simulink model "Cubesat_Control"  (R2023b)
settings: Solver=VariableStepAuto  StartTime=0.0  StopTime=5  FixedStep=1e-3  RelTol=1e-3
values from neighbouring files (symbols this model uses):
  Kd = 1.7377    [Controller_Project.m]
  Kp = 0.026425    [Controller_Project.m]
  Tf = 0.0050352    [Controller_Project.m]
libraries: slpidlib x1, spspowerguiLib x1
settings Model: Creator=Lucas  LastModifiedBy=Lucas

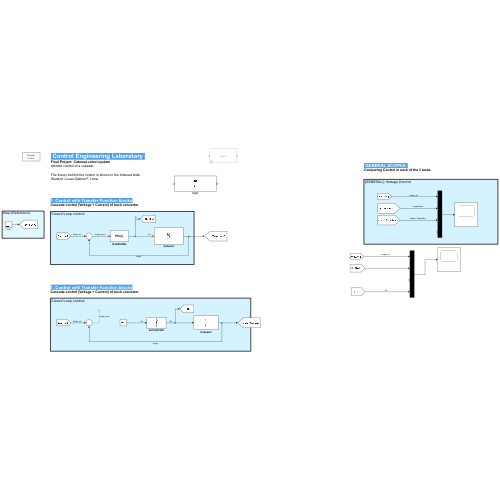
[thumbnail: Simulink's stored preview of the top-level diagram]
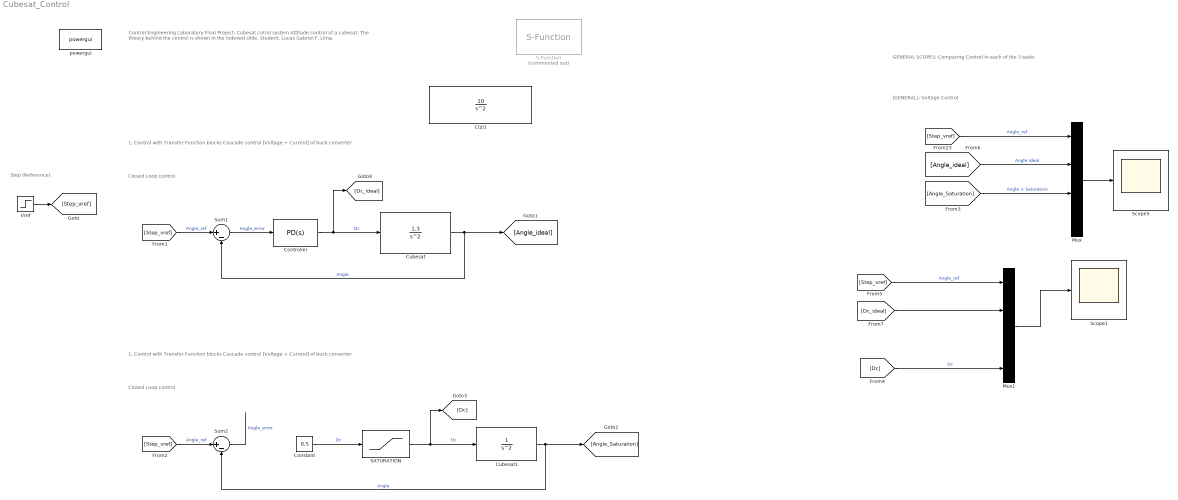
== system Cubesat_Control ==
  note: GENERAL SCOPES:
      | Comparing Control in each of the 3 tasks
  note: [GENERAL]: Voltage Control
  note: Closed Loop control
  note: 1. Control with Transfer Function blocks
      | Cascade control [Voltage + Current] of buck converter
  note: Step (Reference)
  note: Control Engineering Laboratory
      | Final Project: Cubesat cotrol system
      | Attitude control of a cubesat.
      |
      | The theory behind the control is shown in the indexed slide.
      | Student: Lucas Gabriel F. Lima.
  note: 1. Control with Transfer Function blocks
      | Cascade control [Voltage + Current] of buck converter
  note: Closed Loop control
  C(z)1 : TransferFcn  Numerator=[10]  Denominator=[1,0 , 0]
  Constant : Constant  Value=0.5
  Controller : slpidlib/PID Controller  Controller=PD  Form=Parallel  TimeDomain=Continuous-time  UseExternalTs=off  SampleTime=0.001  IntegratorMethod=Forward Euler  FilterMethod=Forward Euler  ControllerParametersSource=internal  P=Kp  I=0.050703  UseKiTs=off  D=Kd  N=1/Tf  UseFilter=on  TunerSelectOption=Transfer Function Based (PID Tuner App)  InitialConditionSource=internal  InitialConditionForIntegrator=0  InitialConditionForFilter=0  DifferentiatorICPrevScaledInput=0  ExternalReset=none  TrackingMode=off  Kt=1  LimitOutput=off  SatLimitsSource=internal  UpperSaturationLimit=inf  LowerSaturationLimit=-inf  LinearizeAsGain=on  AntiWindupMode=none  Kb=1  LimitIntegrator=off  UpperIntegratorSaturationLimit=inf  LowerIntegratorSaturationLimit=-inf  POutMin=[]  POutMax=[]  IOutMin=[]  IOutMax=[]  DOutMin=[]  DOutMax=[]  NOutMin=[]  NOutMax=[]  SumOutMin=[]  SumOutMax=[]  SaturationOutMin=[]  SaturationOutMax=[]  PParamMin=[]  PParamMax=[]  IParamMin=[]  IParamMax=[]  DParamMin=[]  DParamMax=[]  NParamMin=[]  NParamMax=[]  KbParamMin=[]  KbParamMax=[]  KtParamMin=[]  KtParamMax=[]  KbOutMin=[]  KbOutMax=[]  KtOutMin=[]  KtOutMax=[]  IntegratorOutMin=[]  IntegratorOutMax=[]  FilterOutMin=[]  FilterOutMax=[]  SumI1OutMin=[]  SumI1OutMax=[]  SumI2OutMin=[]  SumI2OutMax=[]  SumI3OutMin=[]  SumI3OutMax=[]  SumI4OutMin=[]  SumI4OutMax=[]  SumDOutMin=[]  SumDOutMax=[]  DifferentiatorOutMin=[]  DifferentiatorOutMax=[]  FilterDiffOutCoefMin=[]  FilterDiffOutCoefMax=[]  ReciprocalOutMin=[]  ReciprocalOutMax=[]  SumDenOutMin=[]  SumDenOutMax=[]  SumNumOutMin=[]  SumNumOutMax=[]  DivideOutMin=[]  DivideOutMax=[]  UdiffTsProdOutMin=[]  UdiffTsProdOutMax=[]  NTsProdOutMin=[]  NTsProdOutMax=[]  UintegralTsProdOutMin=[]  UintegralTsProdOutMax=[]  UngainTsProdOutMin=[]  UngainTsProdOutMax=[]  ClampingZeroOutDataTypeStr=Inherit: Inherit via back propagation  ClampingZeroOutMin=[]  ClampingZeroOutMax=[]  FilterDenConstantOutDataTypeStr=Inherit: Inherit via back propagation  FilterDenConstantOutMin=[]  FilterDenConstantOutMax=[]  PCopyOutDataTypeStr=Inherit: Inherit via back propagation  PCopyOutMin=[]  PCopyOutMax=[]  NCopyOutDataTypeStr=Inherit: Inherit via back propagation  NCopyOutMin=[]  NCopyOutMax=[]  IntegratorContinuousStateAttributes=''  IntegratorStateMustResolveToSignalObject=off  IntegratorRTWStateStorageClass=Auto  FilterContinuousStateAttributes=''  FilterStateMustResolveToSignalObject=off  FilterRTWStateStorageClass=Auto  ParallelPVariant=InternalParameters  IdealPVariant=Disabled  IVariant=Disabled  DVariant=InternalParameters  IntegratorVariant=Disabled  SatVariant=Disabled  AWVariant=Disabled  PCopyVariant=Disabled  TRVariant=Disabled  FdbkBlocksVariant=Forward  IdealPFdbkVariant=Disabled  SatFdbkVariant=Disabled  DerivativeFilterVariant=ContFilter  NVariant=InternalParameters  NCopyVariant=Disabled  FilterICVariant=InternalICsFilter  IntegratorICVariant=Disabled  ExternalResetVariant=Disabled  TRSumVariant=Passthrough  SumFdbkVariant=Disabled  SumVariant=Sum_PD  TsampFilterVariant=InternalTs  TsampNgainVariant=Passthrough  TsampIntegralVariant=Disabled_SignalSpec  ExternalSaturationOutDataTypeStr=Inherit: Same as second input
  Cubesat : TransferFcn  Numerator=[1.3]  Denominator=[1,0 , 0]
  Cubesat1 : TransferFcn  Denominator=[1,0 , 0]
  Mux : Mux
  Mux1 : Mux
  S-Function : S-Function  Commented=on  SFunctionDeploymentMode=off  EnableBusSupport=off
  SATURATION : Saturate
  Scope1 : Scope
  Scope5 : Scope
  Sum1 : Sum  Inputs=|+-
  Sum2 : Sum  Inputs=|+-
  Vref : Step  Time=0  After=90  SampleTime=0
  powergui : spspowerguiLib/powergui  Priority=1  SimulationMode=Discrete  SampleTime=1e-8  frequency=60  Iterations=50  frequencyindice=0  Pbase=100e6  ErrMax=1e-4  UnitsV=kV  UnitsW=MW  buscounter=0  FunctionMessages=off  echomessages=off  EnableUseOfTLC=off  CurrentSourceSwitches=off  DisableSnubberDevices=off  DisableRonSwitches=off  DisableVfSwitches=off  DisplayEquations=off  AutomaticDiscreteSolvers=off  SolverType=Tustin/Backward Euler (TBE)  Interpol=off  ExternalGateDelay=off  methode=off  Ts=100  x0status=blocks  SPID=on  SwTol=0  HookPort=off  NonlinearTolerance=1e-4  nMaxIteration=100  ContinueOnMaxIteration=off  RestoreLinks=warning  ResistiveCurrentMeasurement=off  Frange=[0:2:500]  Ylog=off  Xlog=on  ShowGrid=off  save=off  variable=ZData  structure=0  ZoomFFT=off  StartTime=0.0  cycles=1  DisplayStyle=1  fundamental=60  FreqAxis=off  MaxFrequency=1000  frequencyindicesteady=1  RmsSteady=1  display=off
  wires:
  [Step_vref] -> Mux/1  "Angle_ref"
  Mux/1 -> Scope5/1
  [Angle_ideal] -> Mux/2  "Angle Ideal"
  [Step_vref] -> Sum1/1  "Angle_ref"
  Controller/1 -> [Dc_ideal], Cubesat/1  "Dc"
  Sum1/1 -> Controller/1  "Angle_error"
  Cubesat/1 -> [Angle_ideal], Sum1/2  "Angle"
  Vref/1 -> [Step_vref]
  [Dc] -> Mux1/4  "Dc"
  [Step_vref] -> Mux1/1  "Angle_ref"
  Mux1/1 -> Scope1/1
  Constant/1 -> SATURATION/1  "Dc"
  Cubesat1/1 -> [Angle_Saturation], Sum2/2  "Angle"
  Sum2/1 -> ?  "Angle_error"
  [Step_vref] -> Sum2/1  "Angle_ref"
  SATURATION/1 -> [Dc], Cubesat1/1  "Dc"
  [Angle_Saturation] -> Mux/3  "Angle + Saturation"
  [Dc_ideal] -> Mux1/2
